simulink model "Trajectorygenerator_Ctc"  (R2017b)
settings: Solver=ode2  StartTime=0.0  StopTime=12  FixedStep=0.001  RelTol=1e-3
values from neighbouring files (symbols this model uses):
  kuk = SerialLink(L)    [Preload.m]    (also in PreloadTest.m)
undefined symbols (not defined in the file or in its folder): jacky, jackydot
settings Model: Creator=mkiri  LastModifiedBy=mkiri

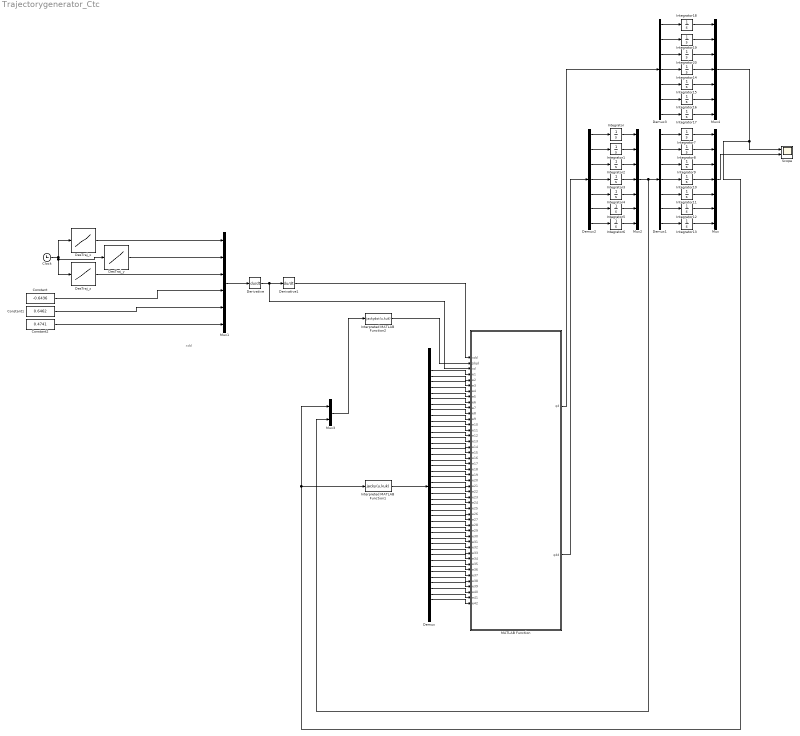
== system Trajectorygenerator_Ctc ==
  note: xdd
  Clock : Clock
  Constant : Constant  Value=-0.6436
  Constant1 : Constant  Value=0.6462
  Constant2 : Constant  Value=0.4741
  Demux : Demux  Outputs=42
  Demux1 : Demux  Outputs=7
  Demux2 : Demux  Outputs=7
  Demux3 : Demux  Outputs=7
  Derivative : Derivative
  Derivative1 : Derivative
  DesTraj_x : Lookup_n-D  NumberOfTableDimensions=1  BreakpointsForDimension1=[0 5]  Table=[0.2314 0.2314]  ExtrapMethod=Clip  UseLastTableValue=on  InternalRulePriority=Speed  RndMeth=Simplest  InputSameDT=on
  DesTraj_y : Lookup_n-D  NumberOfTableDimensions=1  BreakpointsForDimension1=[0 12]  Table=[-0.2689 0.0689]  ExtrapMethod=Clip  UseLastTableValue=on  InternalRulePriority=Speed  RndMeth=Simplest  InputSameDT=on
  DesTraj_z : Lookup_n-D  NumberOfTableDimensions=1  BreakpointsForDimension1=[0 3 6 9 12]  Table=[0.9093 0.7093 0.9093 0.7093 0.9093]  InterpMethod=Cubic spline  ExtrapMethod=Clip  UseLastTableValue=on  InternalRulePriority=Speed  RndMeth=Simplest  InputSameDT=on
  Integrator{,1..7,18} (9 alike) : Integrator
  Integrator10 : Integrator  InitialCondition=1.57079632679490
  Integrator11 : Integrator  InitialCondition=0.401425727958696
  Integrator12 : Integrator  InitialCondition=0.157079632679490
  Integrator13 : Integrator  InitialCondition=0.139626340159546
  Integrator14 : Integrator  InitialCondition=1.57079632679490
  Integrator15 : Integrator  InitialCondition=0.401425727958696
  Integrator16 : Integrator  InitialCondition=0.157079632679490
  Integrator17 : Integrator  InitialCondition=0.139626340159546
  Integrator19 : Integrator  InitialCondition=0.436332312998582
  Integrator20 : Integrator  InitialCondition=-0.523598775598299
  Integrator8 : Integrator  InitialCondition=0.436332312998582
  Integrator9 : Integrator  InitialCondition=-0.523598775598299
  Interpreted MATLAB Function1 : MATLABFcn  MATLABFcn=jacky(u,kuk)
  Interpreted MATLAB Function2 : MATLABFcn  MATLABFcn=jackydot(u,kuk)
  MATLAB Function : MATLAB Function  TreatAsAtomicUnit=on
  Mux : Mux  Inputs=7
  Mux1 : Mux  Inputs=6
  Mux2 : Mux  Inputs=7
  Mux3 : Mux  Inputs=2
  Mux4 : Mux  Inputs=7
  Scope : Scope  NumInputPorts=2
  wires:
  Clock/1 -> DesTraj_y/1, DesTraj_z/1, DesTraj_x/1
  DesTraj_y/1 -> Mux1/2
  DesTraj_x/1 -> Mux1/1
  DesTraj_z/1 -> Mux1/3
  Demux/27 -> MATLAB Function/30(e27)
  Demux/16 -> MATLAB Function/19(e16)
  Interpreted MATLAB Function1/1 -> Demux/1
  Demux/17 -> MATLAB Function/20(e17)
  Mux4/1 -> Interpreted MATLAB Function1/1, Mux3/1, Scope/1
  Demux/18 -> MATLAB Function/21(e18)
  Demux/9 -> MATLAB Function/12(e9)
  Demux/29 -> MATLAB Function/32(e29)
  Demux/19 -> MATLAB Function/22(e19)
  Demux/21 -> MATLAB Function/24(e21)
  Demux/11 -> MATLAB Function/14(e11)
  Demux/14 -> MATLAB Function/17(e14)
  Demux/23 -> MATLAB Function/26(e23)
  Demux/20 -> MATLAB Function/23(e20)
  Demux/6 -> MATLAB Function/9(e6)
  Demux/28 -> MATLAB Function/31(e28)
  Demux/15 -> MATLAB Function/18(e15)
  Demux/4 -> MATLAB Function/7(e4)
  Demux/33 -> MATLAB Function/36(e33)
  Demux/5 -> MATLAB Function/8(e5)
  Demux/25 -> MATLAB Function/28(e25)
  Demux/8 -> MATLAB Function/11(e8)
  Demux/12 -> MATLAB Function/15(e12)
  Demux/26 -> MATLAB Function/29(e26)
  Demux/37 -> MATLAB Function/40(e37)
  Demux/34 -> MATLAB Function/37(e34)
  Demux/7 -> MATLAB Function/10(e7)
  Demux/24 -> MATLAB Function/27(e24)
  Demux/30 -> MATLAB Function/33(e30)
  Demux/22 -> MATLAB Function/25(e22)
  Demux/10 -> MATLAB Function/13(e10)
  Demux/3 -> MATLAB Function/6(e3)
  Demux/31 -> MATLAB Function/34(e31)
  Demux/40 -> MATLAB Function/43(e40)
  Demux/35 -> MATLAB Function/38(e35)
  Demux/1 -> MATLAB Function/4(e1)
  Demux/42 -> MATLAB Function/45(e42)
  Demux/2 -> MATLAB Function/5(e2)
  Demux/39 -> MATLAB Function/42(e39)
  Demux/13 -> MATLAB Function/16(e13)
  Demux/36 -> MATLAB Function/39(e36)
  Demux/32 -> MATLAB Function/35(e32)
  Demux/41 -> MATLAB Function/44(e41)
  Demux/38 -> MATLAB Function/41(e38)
  Integrator13/1 -> Mux/7
  Integrator12/1 -> Mux/6
  Integrator10/1 -> Mux/4
  Integrator9/1 -> Mux/3
  Integrator8/1 -> Mux/2
  Integrator7/1 -> Mux/1
  Integrator11/1 -> Mux/5
  Interpreted MATLAB Function2/1 -> MATLAB Function/2(Jdqd)
  Mux1/1 -> Derivative/1
  Integrator4/1 -> Mux2/5
  Integrator/1 -> Mux2/1
  Integrator1/1 -> Mux2/2
  Integrator2/1 -> Mux2/3
  Integrator3/1 -> Mux2/4
  Integrator5/1 -> Mux2/6
  Integrator6/1 -> Mux2/7
  Mux2/1 -> Mux3/2, Demux1/1
  Demux1/1 -> Integrator7/1
  Demux1/2 -> Integrator8/1
  Demux1/3 -> Integrator9/1
  Demux1/4 -> Integrator10/1
  Demux1/5 -> Integrator11/1
  Demux1/7 -> Integrator13/1
  Demux1/6 -> Integrator12/1
  Mux3/1 -> Interpreted MATLAB Function2/1
  MATLAB Function/2(qdd) -> Demux2/1
  Demux2/6 -> Integrator5/1
  Demux2/7 -> Integrator6/1
  Demux2/5 -> Integrator4/1
  Demux2/4 -> Integrator3/1
  Demux2/3 -> Integrator2/1
  Demux2/2 -> Integrator1/1
  Demux2/1 -> Integrator/1
  Constant1/1 -> Mux1/5
  Constant2/1 -> Mux1/6
  Constant/1 -> Mux1/4
  Derivative1/1 -> MATLAB Function/1(xdd)
  Derivative/1 -> MATLAB Function/3(xd), Derivative1/1
  Demux3/6 -> Integrator16/1
  Demux3/7 -> Integrator17/1
  Demux3/5 -> Integrator15/1
  Demux3/4 -> Integrator14/1
  Demux3/3 -> Integrator20/1
  Demux3/2 -> Integrator19/1
  Demux3/1 -> Integrator18/1
  MATLAB Function/1(qd) -> Demux3/1
  Integrator15/1 -> Mux4/5
  Integrator18/1 -> Mux4/1
  Integrator19/1 -> Mux4/2
  Integrator20/1 -> Mux4/3
  Integrator14/1 -> Mux4/4
  Integrator16/1 -> Mux4/6
  Integrator17/1 -> Mux4/7
  Mux/1 -> Scope/2

== matlab function Trajectorygenerator_Ctc/MATLAB Function ==
  data: qd output; xdd input; qdd output; Jdqd input; xd input; e1 input; e2 input; e3 input; e4 input; e5 input; e6 input; e7 input; e8 input; e9 input; e10 input; e11 input; e12 input; e13 input; e14 input; e15 input; e16 input; e17 input; e18 input; e19 input; e20 input; e21 input; e22 input; e23 input; e24 input; e25 input; e26 input; e27 input; e28 input; e29 input; e30 input; e31 input; e32 input; e33 input; e34 input; e35 input; e36 input; e37 input; e38 input; e39 input; e40 input; e41 input; e42 input
function [qd,qdd]  = fcn(xdd,Jdqd,xd,e1,e2,e3,e4,e5,e6,e7,e8,e9,e10,e11,e12,e13,e14,e15,e16,e17,e18,e19,e20,e21,e22,e23,e24,e25,e26,e27,e28,e29,e30,e31,e32,e33,e34,e35,e36,e37,e38,e39,e40,e41,e42)

J = [e1	e7	e13	e19	e25	e31	e37
e2	e8	e14	e20	e26	e32	e38
e3	e9	e15	e21	e27	e33	e39
e4	e10	e16	e22	e28	e34	e40
e5	e11	e17	e23	e29	e35	e41
e6	e12	e18	e24	e30	e36	e42];
%Js = J((1):(3),(1):(7));

qdd = pinv(J)*(xdd-Jdqd);
qd = pinv(J)*(xd);
